simulink model "ukol_2_model"  (R2017a)
settings: Solver=VariableStepAuto  StartTime=0.0  StopTime=100  MaxStep=1e-2  RelTol=1e-3
values from neighbouring files (symbols this model uses):
  K = tf([kritickeK], [1])    [LSbod2a.m]    (also in ukol_1_a_script.m = 5; ukol_2_a_script.m = 7.16143410213; ukol_2_c_script.m = 0.9 * K_krit; ukol_5_script.m = [k1 k2]')
libraries: cstblocks x1
settings Model: Creator=tomas  LastModifiedBy=tomas

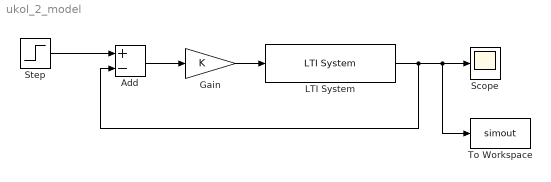
== system ukol_2_model ==
  Add : Sum  Inputs=+-
  Gain : Gain  Gain=K
  LTI System : cstblocks/LTI System  sys=Fs_servo  IC=[]
  Scope : Scope
  Step : Step  SampleTime=0
  To Workspace : ToWorkspace  VariableName=simout  SaveFormat=Timeseries  SampleTime=-1
  wires:
  Gain/1 -> LTI System/1
  LTI System/1 -> Add/2, To Workspace/1, Scope/1
  Add/1 -> Gain/1
  Step/1 -> Add/1
